simulink model "MLIB_VSub_BAM"  (Simulink 9.3)
settings: Solver=VariableStepAuto  StartTime=0.0  StopTime=10.0  RelTol=1e-3
settings Model: Creator=nxf41029  LastModifiedBy=nxf41029
settings DataIOCC: SaveFormat=Dataset  SignalLoggingSaveFormat=Dataset  ReturnWorkspaceOutputs=on
settings OptimizationCC: LifeSpan=auto
settings DebuggingCC: UnderspecifiedInitializationDetection=Simplified  MergeDetectMultiDrivingBlocksExec=error  FcnCallInpInsideContextMsg=error  SFUnexpectedBacktrackingDiag=error  SFNoUnconditionalDefaultTransitionDiag=error  SFExecutionAtInitializationDiag=warning  ArithmeticOperatorsInVariantConditions=error
settings HardwareCC: ProdBitPerPointer=64  ProdBitPerSizeT=64  ProdBitPerPtrDiffT=64  ProdLargestAtomicFloat=Float  ProdIntDivRoundTo=Zero  ProdEndianess=LittleEndian  ProdWordSize=64  ProdHWDeviceType=Intel->x86-64 (Windows64)
settings ModelReferenceCC: PropagateSignalLabelsOutOfModel=on
settings SFSimCC: SimUseLocalCustomCode=on
settings RTWCC: RTWUseLocalCustomCode=on
settings CodeAppCC: StateflowObjectComments=off
settings GRTTargetCC: TargetLangStandard=C99 (ISO)  CombineOutputUpdateFcns=on  GRTInterface=off
settings ConfigComp: CovMetricSettings=dwe  CovHtmlReporting=off  CovSaveCumulativeToWorkspaceVar=off  CovSaveSingleToWorkspaceVar=off  CovExternalEMLEnable=on

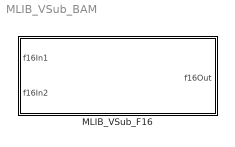
== system MLIB_VSub_BAM ==
  MLIB_VSub_F16 : Subsystem  TreatAsAtomicUnit=on  mask(MLIB_VSub_F16){}
      mask help: Vector substraction in 16-bit fixed-point fractional implementation.
      mask init:
      | if ~evalin('base','exist(''tS8'',''var'')')
      |   if (2 ~= exist('SWLIBS_Typedefs.mat','file'))
      |       error('File SWLIBS_Typedefs.mat is not on the Matlab path. Please add the AMMCLIB "bam" folder in the Matlab Search Path.');
      |   else
      |       evalin('base', 'load(''SWLIBS_Typedefs.mat'')');
      |   end
      | end
      settings: RTWSystemCode=Inline
      mask Display: pos = get_param(gcb, 'Position');width = pos(3) - pos(1); height = pos(4) - pos(2);tX=width/2;tY=height - 8;color('black');text(tX,tY, 'MLIB_VSub_F16', 'horizontalAlignment', 'center');

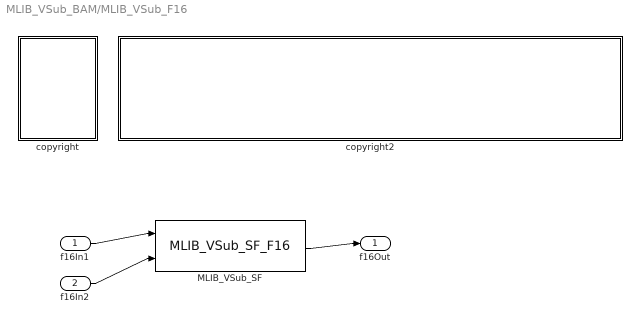
== system MLIB_VSub_BAM/MLIB_VSub_F16 ==
  f16In1 : Inport  OutDataTypeStr=Bus: SWLIBS_2Syst_F16  BusOutputAsStruct=on
  f16In2 : Inport  Port=2  OutDataTypeStr=Bus: SWLIBS_2Syst_F16  BusOutputAsStruct=on
  MLIB_VSub_SF : S-Function  FunctionName=MLIB_VSub_SF_F16  SFunctionDeploymentMode=off  EnableBusSupport=off
  copyright : Subsystem
      mask Display: text(10,90,'FILE:');text(10,75,'DESRIPTION:');text(10,60,'COPYRIGHT:');text(10,45,'VERSION:');text(10,30,'DATE:')
  copyright2 : Subsystem
      mask Display: text(10,90,'MLIB_VSub_BAM_F16.mdl');text(10,75,'Vector substraction.');text(10,60,'NXP 2020');text(10,45,'1.0');text(10,30,'01-Jun-2020');
  f16Out : Outport
  wires:
  f16In1/1 -> MLIB_VSub_SF/1
  f16In2/1 -> MLIB_VSub_SF/2
  MLIB_VSub_SF/1 -> f16Out/1

== system MLIB_VSub_BAM/MLIB_VSub_F16/copyright ==

== system MLIB_VSub_BAM/MLIB_VSub_F16/copyright2 ==
